simulink model "modulation"  (R2014a)
settings: Solver=ode45  StartTime=0.0  StopTime=10.0  RelTol=1e-3
settings Model: Creator=HEWLETT PACKARD  LastModifiedBy=HEWLETT PACKARD

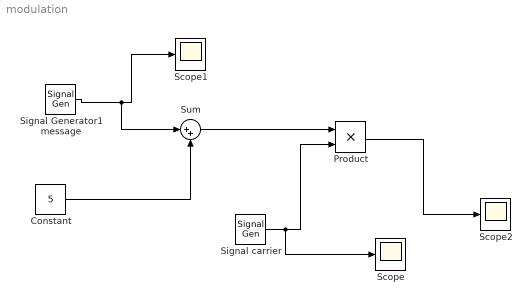
== system modulation ==
  Constant : Constant  Value=5
  Product : Product
  Scope : Scope
  Scope1 : Scope
  Scope2 : Scope
      settings: SaveName=ScopeData2
  "Signal carrier " : SignalGenerator  Amplitude=10  Frequency=30  Units=rad/sec
  Signal Generator1 message : SignalGenerator  Amplitude=5  Frequency=30  Units=rad/sec
  Sum : Sum  Inputs=|++
  wires:
  Signal Generator1 message/1 -> Sum/1, Scope1/1
  Sum/1 -> Product/1
  Constant/1 -> Sum/2
  "Signal carrier "/1 -> Scope/1, Product/2
  Product/1 -> Scope2/1
